simulink model "nonlinear_lqr"  (R2021a)
settings: Solver=VariableStepAuto  StartTime=0.0  StopTime=100.0  RelTol=1e-3
undefined symbols (not defined in the file): K
settings Model: Creator=savna  LastModifiedBy=savna

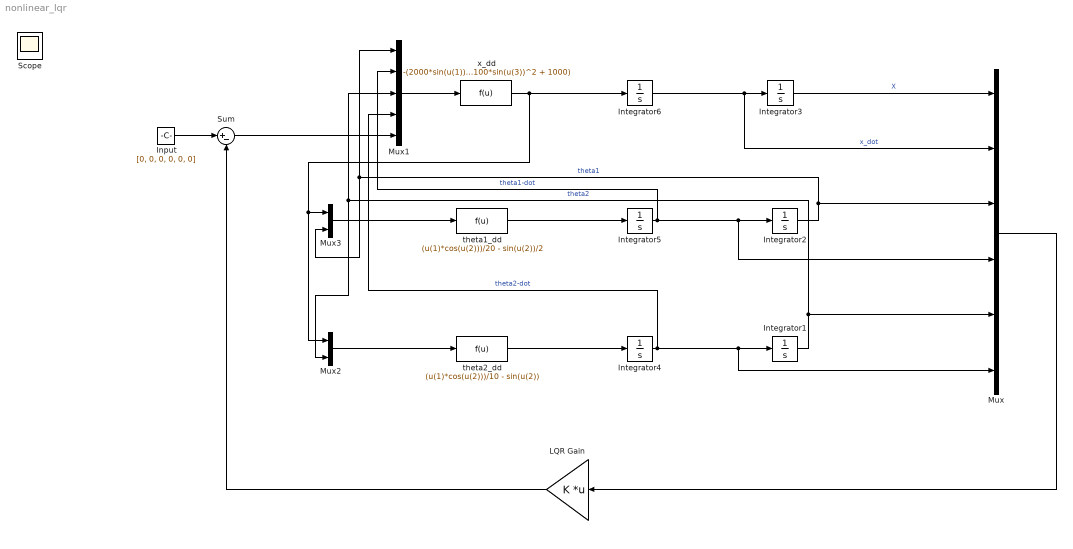
== system nonlinear_lqr ==
  Input : Constant  Value=[0, 0, 0, 0, 0, 0]
  Integrator1 : Integrator  InitialCondition=0.1
  Integrator2 : Integrator  InitialCondition=0.1
  Integrator3 : Integrator  InitialCondition=0.5
  Integrator4 : Integrator
  Integrator5 : Integrator
  Integrator6 : Integrator
  LQR Gain : Gain  Gain=K  Multiplication=Matrix(K*u)
  Mux : Mux  Inputs=6
  Mux1 : Mux  Inputs=5
  Mux2 : Mux  Inputs=2
  Mux3 : Mux  Inputs=2
  Sum : Sum  Inputs=|+-
  theta1_dd : Fcn  Expr=(u(1)*cos(u(2)))/20 - sin(u(2))/2
  theta2_dd : Fcn  Expr=(u(1)*cos(u(2)))/10 - sin(u(2))
  x_dd : Fcn  Expr=-(2000*sin(u(1))*u(2)^2 + 1000*sin(u(3))*u(4)^2 - u(5) + 1000*cos(u(1))*sin(u(1)) - 1000*cos(u(3))*sin(u(3)))/(100*sin(u(1))^2 + 100*sin(u(3))^2 + 1000)
  Scope : Scope
  wires:
  Integrator3/1 -> Mux/1  "X"
  Integrator6/1 -> Mux/2, Integrator3/1  "x_dot"
  Mux/1 -> LQR Gain/1
  LQR Gain/1 -> Sum/2
  Sum/1 -> Mux1/5
  Mux1/1 -> x_dd/1
  Mux2/1 -> theta2_dd/1
  Mux3/1 -> theta1_dd/1
  Integrator4/1 -> Mux1/4, Integrator1/1, Mux/6  "theta2-dot"
  Integrator1/1 -> Mux2/2, Mux1/3, Mux/5  "theta2"
  x_dd/1 -> Mux2/1, Mux3/1, Integrator6/1
  theta2_dd/1 -> Integrator4/1
  Integrator5/1 -> Mux1/2, Mux/4, Integrator2/1  "theta1-dot"
  theta1_dd/1 -> Integrator5/1
  Integrator2/1 -> Mux3/2, Mux1/1, Mux/3  "theta1"
  Input/1 -> Sum/1
